simulink model "accelSim"  (R2025a)
settings: Solver=VariableStepAuto  StartTime=0.0  StopTime=5  RelTol=1e-3
InitFcn:
  | init_params();
libraries: simulink x2
settings Model: Creator=PC5  LastModifiedBy=PC5

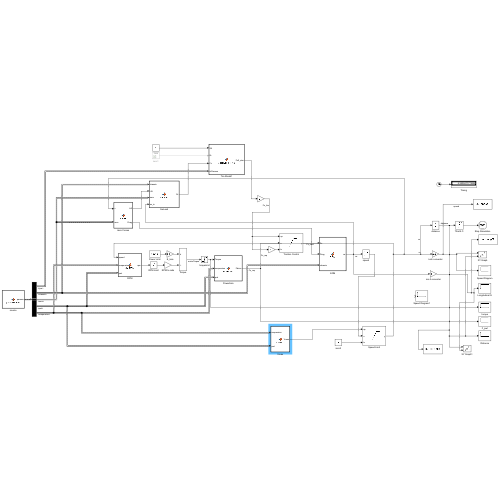
[thumbnail: Simulink's stored preview of the top-level diagram]
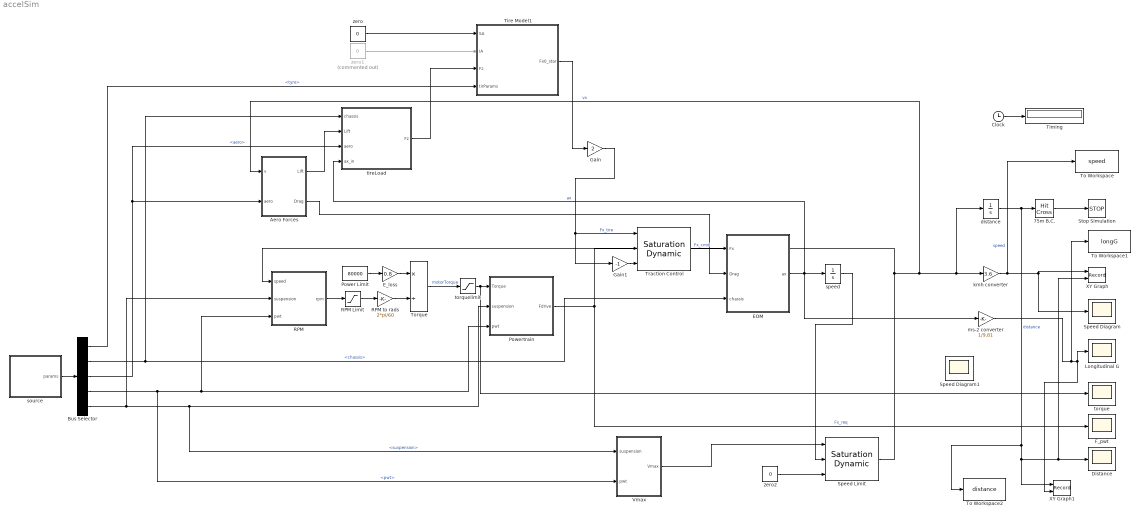
== system accelSim ==
  75m B.C. : HitCross  HitCrossingOffset=75  HitCrossingDirection=rising
  Aero Forces : MATLAB Function  TreatAsAtomicUnit=on
  Bus Selector : BusSelector  OutputSignals=tyre,chassis,aero,pwt,suspension
  Clock : Clock
  Distance : Scope
      settings: ActiveDisplayYMinimum=-1  ActiveDisplayYMaximum=1
  EOM : MATLAB Function  TreatAsAtomicUnit=on
  E_loss : Gain  Gain=0.8
  F_pwt : Scope
      settings: ActiveDisplayYMinimum=-1  ActiveDisplayYMaximum=1  DataLoggingVariableName=ScopeData4
  Gain : Gain  Gain=2
  Gain1 : Gain  Gain=-1
  Longitudinal G : Scope
      settings: Title=Longitudinal Acceleration  ActiveDisplayYMinimum=0  ActiveDisplayYMaximum=1.229  YLabel=Acceleration (G)  DataLoggingVariableName=ScopeData2
  Power Limit : Constant  Value=80000
  Powertrain : MATLAB Function  TreatAsAtomicUnit=on
  RPM : MATLAB Function  TreatAsAtomicUnit=on
  RPM Limit : Saturate  UpperLimit=10000  LowerLimit=0
  RPM to rads : Gain  Gain=2*pi/60
  Speed Diagram : Scope
      settings: ActiveDisplayYMinimum=-46.787279137521928  ActiveDisplayYMaximum=222.55498688416193
  Speed Diagram1 : Scope
      settings: ActiveDisplayYMinimum=-46.787279137521928  ActiveDisplayYMaximum=222.55498688416193  DataLoggingVariableName=ScopeData3
  Speed Limit : simulink/Discontinuities/Saturation Dynamic  OutMin=[]  OutMax=[]  OutDataTypeStr=Inherit: Same as second input  OutDataType=fixdt(1, 16)  OutScaling=2^-10  DoSatur=off
  Stop Simulation : Stop
  Timing : Display
  Tire Model1 : MATLAB Function  TreatAsAtomicUnit=on
  To Workspace : ToWorkspace  VariableName=speed  SaveFormat=Timeseries  SampleTime=-1
  To Workspace1 : ToWorkspace  VariableName=longG  SaveFormat=Timeseries  SampleTime=-1
  To Workspace2 : ToWorkspace  VariableName=distance  SaveFormat=Timeseries  SampleTime=-1
  Torque : Product  Inputs=*/  InputSameDT=on  OutMin=0  OutMax=300
  Traction Control : simulink/Discontinuities/Saturation Dynamic  OutMin=[]  OutMax=[]  OutDataTypeStr=Inherit: Same as second input  OutDataType=fixdt(1, 16)  OutScaling=2^-10  DoSatur=off
  Vmax : MATLAB Function  TreatAsAtomicUnit=on
  XY Graph : Record  NumPorts=2.0  FileSettingsInternal="{\"entries\":[{\"content\":{\"excelSettings\":{\"content\":{},\"type\":\"Streamout.ExcelSettings\"},\"parquetSettings\":{\"content\":{},\"type\":\"Streamout.ParquetSettings\"}},\"type\":\"Streamout.FileSettingStorage\",\"uuid\":\"\"}],\"packageUris\":[\"http:\\/\\/schema.mathworks.com\\/mf0\\/streamout_blocks\\/R2020a\"],\"version\":\"1.0\"}"  FrameSettings=[0, 0]  Layout=[1 1]  SignalsInternal="{\"entries\":[{\"content\":{\"signals\":[{\"content\":{\"blockPath\":[],\"dimensions\":[1],\"domain\":\"\",\"lineColor\":\"#a2142f\",\"plots\":[ 1 ],\"port\":1,\"sid\":[\"\"],\"signalID\":1,\"signalName\":\"speed\"},\"type\":\"RecordBlkView.Signal\",\"uuid\":\"\"},{\"content\":{\"blockPath\":[],\"dimensions\":[1],\"domain\":\"\",\"lineColor\":\"#139fff\",\"plots\":[ 1 ],\"port\":2,\"sid\":[\"\"],\"signalID\":2,\"signalName\":\"distance\"},\"type\":\"RecordBlkView.Signal\",\"uuid\":\"\"}]},\"type\":\"RecordBlkView.InputSignals\",\"uuid\":\"\"}],\"packageUris\":[\"http:\\/\\/schema.mathworks.com\\/mf0\\/streamout_blocks\\/R2020a\"],\"version\":\"1.0\"}"  VisualizationBindings="{\"xyplotplugin\":{\"info\":[{\"series\":[{\"bindingParametersList\":[{\"parameter\":\"X-Axis\",\"signalID\":1,\"signalName\":\"speed\"},{\"parameter\":\"Y-Axis\",\"signalID\":2,\"signalName\":\"distance\"}],\"seriesID\":0}],\"subplotID\":1}]}}"  CompatibilityTag=XY
  XY Graph1 : Record  NumPorts=2.0  FileSettingsInternal="{\"entries\":[{\"content\":{\"excelSettings\":{\"content\":{},\"type\":\"Streamout.ExcelSettings\"},\"parquetSettings\":{\"content\":{},\"type\":\"Streamout.ParquetSettings\"}},\"type\":\"Streamout.FileSettingStorage\",\"uuid\":\"\"}],\"packageUris\":[\"http:\\/\\/schema.mathworks.com\\/mf0\\/streamout_blocks\\/R2020a\"],\"version\":\"1.0\"}"  FrameSettings=[0, 0]  Layout=[1 1]  SignalsInternal="{\"entries\":[{\"content\":{\"signals\":[{\"content\":{\"blockPath\":[],\"dimensions\":[1],\"domain\":\"\",\"lineColor\":\"#a2142f\",\"plots\":[ 1 ],\"port\":1,\"sid\":[\"\"],\"signalID\":1,\"signalName\":\"distance\"},\"type\":\"RecordBlkView.Signal\",\"uuid\":\"\"},{\"content\":{\"blockPath\":[],\"dimensions\":[1],\"domain\":\"\",\"lineColor\":\"#139fff\",\"plots\":[ 1 ],\"port\":2,\"sid\":[\"\"],\"signalID\":2,\"signalName\":\"ms-2 converter\"},\"type\":\"RecordBlkView.Signal\",\"uuid\":\"\"}]},\"type\":\"RecordBlkView.InputSignals\",\"uuid\":\"\"}],\"packageUris\":[\"http:\\/\\/schema.mathworks.com\\/mf0\\/streamout_blocks\\/R2020a\"],\"version\":\"1.0\"}"  VisualizationBindings="{\"xyplotplugin\":{\"info\":[{\"series\":[{\"bindingParametersList\":[{\"parameter\":\"X-Axis\",\"signalID\":1,\"signalName\":\"distance\"},{\"parameter\":\"Y-Axis\",\"signalID\":2,\"signalName\":\"ms-2 converter\"}],\"seriesID\":0}],\"subplotID\":1}]}}"  CompatibilityTag=XY
  distance : Integrator
  kmh converter : Gain  Gain=3.6
  ms-2 converter : Gain  Gain=1/9.81
  source : MATLAB Function  TreatAsAtomicUnit=on
  speed : Integrator  LimitOutput=on  LowerSaturationLimit=0
  tireLoad : MATLAB Function  TreatAsAtomicUnit=on
  torque : Scope
      settings: ActiveDisplayYMinimum=122.82034534657527  ActiveDisplayYMaximum=241.9088505170472  DataLoggingVariableName=ScopeData5
  torquelimit : Saturate  UpperLimit=230  LowerLimit=0
  zero : Constant  Value=0
  zero1 : Constant  Commented=on  Value=0
  zero2 : Constant  Value=0
  wires:
  Aero Forces/1(Lift) -> tireLoad/2(Lift)
  Aero Forces/2(Drag) -> EOM/2(Drag)
  EOM/1(ax) -> speed/1, ms-2 converter/1, tireLoad/4(ax_in)  "ax"
  Speed Limit/1 -> distance/1, kmh converter/1, Aero Forces/1(v), RPM/1(speed)  "vx"
  Power Limit/1 -> E_loss/1
  RPM/1(rpm) -> RPM Limit/1
  distance/1 -> 75m B.C./1, To Workspace2/1, XY Graph1/1, XY Graph/2, Distance/1  "distance"
  75m B.C./1 -> Stop Simulation/1
  source/1(params) -> Bus Selector/1
  RPM Limit/1 -> RPM to rads/1
  Powertrain/1(Fdrive) -> Traction Control/2, F_pwt/1  "Fx_req"
  Gain/1 -> Gain1/1, Traction Control/1  "Fx_tire"
  Gain1/1 -> Traction Control/3
  Traction Control/1 -> EOM/1(Fx)  "Fx_cmd"
  Bus Selector/2 -> EOM/3(chassis), tireLoad/1(chassis)  "<chassis>"
  Bus Selector/3 -> Aero Forces/2(aero), tireLoad/3(aero)  "<aero>"
  Bus Selector/4 -> Vmax/2(pwt), Powertrain/3(pwt), RPM/3(pwt)  "<pwt>"
  Bus Selector/5 -> Vmax/1(suspension), Powertrain/2(suspension), RPM/2(suspension)  "<suspension>"
  kmh converter/1 -> Speed Diagram/1, XY Graph/1, To Workspace/1  "speed"
  ms-2 converter/1 -> To Workspace1/1, XY Graph1/2, Longitudinal G/1
  RPM to rads/1 -> Torque/2
  torquelimit/1 -> torque/1, Powertrain/1(Torque)
  Torque/1 -> torquelimit/1  "motorTorque"
  Clock/1 -> Timing/1
  zero/1 -> Tire Model1/1(SA)
  zero1/1 -> Tire Model1/2(IA)
  tireLoad/1(Fz) -> Tire Model1/3(Fz)
  Bus Selector/1 -> Tire Model1/4(tirParams)  "<tyre>"
  Tire Model1/1(Fx0_star) -> Gain/1
  E_loss/1 -> Torque/1
  speed/1 -> Speed Limit/2
  zero2/1 -> Speed Limit/3
  Vmax/1(Vmax) -> Speed Limit/1

== matlab function accelSim/Vmax ==
  data: Vmax output; suspension input; pwt input
% calculates aerodynamics

function Vmax  = findmaxv(suspension,pwt)

Vmax = (2*pi/60)*(pwt.max_rpm/pwt.FDR)*suspension.R;



end

== matlab function accelSim/Aero Forces ==
  data: Lift output; Drag output; v input; aero input
% calculates aerodynamics

function [Lift, Drag] = aeroF(v,aero)

Lift = 0.5*aero.farea*aero.CLs*aero.den*v^2;
Drag = 0.5*aero.farea*aero.CDs*aero.den*v^2;


end

== matlab function accelSim/tireLoad ==
  data: chassis input; Lift input; Fz output; aero input; ax_in input
function Fz = tireLoad(chassis,Lift,aero,ax_in)

mass = chassis.car+chassis.driver;
ab = aero.ab_s;
cg_h = chassis.cg_h;
wheelbase = chassis.wheelbase;

% normal load by mass
Fz = (mass*9.81)/4;
% aero downforce
AeroR = Lift*(1-ab);
% load transfer
longLT = Fz*(ax_in/9.81)*cg_h/wheelbase;
% wheel loads per wheel
Fz= Fz+AeroR/2+longLT/2;

end

== matlab function accelSim/EOM ==
  data: Fx input; ax output; Drag input; chassis input
function ax  = EOM(Fx,Drag,chassis)
ax = (Fx-Drag)/(chassis.driver+chassis.car);
end

== matlab function accelSim/RPM ==
  data: rpm output; speed input; suspension input; pwt input
function rpm = findRPM(speed,suspension,pwt)
    R = suspension.R;
    FDR = pwt.FDR;
    rpm = speed / (2*pi*R) * 60 * FDR;
end

== matlab function accelSim/Powertrain ==
  data: Torque input; Fdrive output; suspension input; pwt input
function Fdrive  = findFdrive(Torque,suspension,pwt)
R = suspension.R;
FDR = pwt.FDR;
Fdrive = FDR*Torque/R;
end

== matlab function accelSim/Tire Model1 ==
  data: SA input; IA input; Fz input; tirParams input; Fx0_star output
function Fx0_star  = accelLongForce(SA, IA, Fz, tirParams)
    % processing parameters
    Pa      = 62052.8;
    proParams = calculateParams(Fz, Pa, tirParams);

    % find peak longitudinal force
    a       = 0.05;
    d       = 0.45;
    tol     = 1e-7;
    maxIter = 5000;
    [k_star, Fx0_star, iterGold] = goldenSearchMethod(a, d, tol, maxIter, Fz, IA, tirParams, proParams);
end


function [k_star, Fx0_star, iterGold] = goldenSearchMethod(a, d, tol, maxIter, Fz, gamma, tirParams, proParams)
    % Golden ratio coefficient
    alpha = (sqrt(5) - 1) / 2;
    % Initial interior evaluation points
    b = d - alpha * (d - a);
    c = a + alpha * (d - a);
    for k = 1:maxIter
        % Evaluate magic formula longitudinal force at points b and c
        fx1 = Fx0(Fz, b, gamma, tirParams, proParams);
        fxb = fx1.Fx0;
        fx2 = Fx0(Fz, c, gamma, tirParams, proParams);
        fxc = fx2.Fx0;
        % Termination condition: search window sufficiently small
        if abs(b - a) < tol
            break
        end
        % Maximisation step (choose interval that retains the peak)
        if fxb > fxc
            % Peak lies in [a, c]
            d = c;
            c = b;
            b = d - alpha * (d - a);
        else
            % Peak lies in [b, d]
            a = b;
            b = c;
            c = a + alpha * (d - a);
        end
    end
    % Number of iterations used
    iterGold = k;
    % Select final optimum between the two interior candidates
    if fxb > fxc
        k_star   = b;
        Fx0_star = fxb;
    else
        k_star   = c;
        Fx0_star = fxc;
    end
end

function proParams = calculateParams(Fz, Pa, tirParams)
    % tirParams are fitted parameters from TIR file
    V0 = tirParams.LONGVL; %Nominal speed
    pi0	= tirParams.NOMPRES; %Nominal tyre inflation pressure
    Fz0	= tirParams.FNOMIN; %Nominal wheel load
    LFZO = tirParams.LFZO; % Scale factor of nominal (rated) load
    LMUX = tirParams.LMUX; % Scale factor of Fx peak friction coefficient
    LMUY = tirParams.LMUY; % Scale factor of Fy peak friction coefficient

    % Digressive friction factor
    % On Page 179 of the book is suggested Amu = 10, but after
    % comparing the use of the scaling factors against TNO, Amu = 1
    % was giving perfect match
    Amu = 1;
    LMUX_prime = Amu.*LMUX./(1+(Amu-1).*LMUX); % [Eqn (4.E8) Page 179 - Book]
    LMUY_prime = Amu.*LMUY./(1+(Amu-1).*LMUY); % [Eqn (4.E8) Page 179 - Book]

    % Effect of having a tire with a different nominal load
    Fz0_prime =  LFZO.*Fz0; % [Eqn (4.E1) Page 177 - Book]
    % Normalized change in vertical load
    dfz = (Fz - Fz0_prime)./Fz0_prime; % [Eqn (4.E2a) Page 177 - Book]
    % Normalized change in inflation pressure
    dpi = (Pa - pi0)./pi0; % [Eqn (4.E2b) Page 177 - Book]

    epsilon  = 1e-6;
    
    % Pack processed parameters
    proParams.LMUX_prime = LMUX_prime;
    proParams.LMUY_prime = LMUY_prime;
    proParams.Fz0_prime = Fz0_prime;
    proParams.dfz = dfz;
    proParams.dpi = dpi;
    proParams.epsilon = epsilon;
end

function fxOut = Fx0(Fz, kappa, gamma, tirParams, proParams)
    %[SCALING_COEFFICIENTS]
    LCX     = tirParams.LCX ; % Scale factor of Fx shape factor
    LEX  	= tirParams.LEX ; % Scale factor of Fx curvature factor
    LKX  	= tirParams.LKX ; % Scale factor of Fx slip stiffness
    LHX  	= tirParams.LHX ; % Scale factor of Fx horizontal shift
    LVX  	= tirParams.LVX ; % Scale factor of Fx vertical shift
    LMUX    = tirParams.LMUX ; % Scale factor of Fx peak friction coefficient
    LXAL    = tirParams.LXAL ; % Scale factor of alpha influence on Fx

    %[LONGITUDINAL_COEFFICIENTS]
    PCX1  	=  tirParams.PCX1 ; %Shape factor Cfx for longitudinal force
    PDX1  	=  tirParams.PDX1 ; %Longitudinal friction Mux at Fznom
    PDX2  	=  tirParams.PDX2 ; %Variation of friction Mux with load
    PDX3  	=  tirParams.PDX3 ; %Variation of friction Mux with camber squared
    PEX1  	=  tirParams.PEX1 ; %Longitudinal curvature Efx at Fznom
    PEX2  	=  tirParams.PEX2 ; %Variation of curvature Efx with load
    PEX3  	=  tirParams.PEX3 ; %Variation of curvature Efx with load squared
    PEX4  	=  tirParams.PEX4 ; %Factor in curvature Efx while driving
    PKX1  	=  tirParams.PKX1 ; %Longitudinal slip stiffness Kfx./Fz at Fznom
    PKX2  	=  tirParams.PKX2 ; %Variation of slip stiffness Kfx./Fz with load
    PKX3  	=  tirParams.PKX3 ; %Exponent in slip stiffness Kfx./Fz with load
    PHX1  	=  tirParams.PHX1 ; %Horizontal shift Shx at Fznom
    PHX2  	=  tirParams.PHX2 ; %Variation of shift Shx with load
    PVX1  	=  tirParams.PVX1 ; %Vertical shift Svx./Fz at Fznom
    PVX2  	=  tirParams.PVX2 ; %Variation of shift Svx./Fz with load
    PPX1  	=  tirParams.PPX1 ; %linear influence of inflation pressure on longitudinal slip stiffness
    PPX2  	=  tirParams.PPX2 ; %quadratic influence of inflation pressure on longitudinal slip stiffness
    PPX3  	=  tirParams.PPX3 ; %linear influence of inflation pressure on peak longitudinal friction
    PPX4  	=  tirParams.PPX4 ; %quadratic influence of inflation pressure on peak longitudinal friction
    
    %[PROCESSED PARAMETERS]
    dfz = proParams.dfz;
    dpi = proParams.dpi;
    LMUX_prime = proParams.LMUX_prime;
    epsilon = proParams.epsilon;

    zeta1 = 1;

    Cx = PCX1.*LCX; % (> 0) (4.E11)
    mux = (PDX1 + PDX2.*dfz).*(1 + PPX3.*dpi + PPX4.*dpi.^2).*(1 - PDX3.*gamma.^2).*LMUX; % (4.E13)
    mux(Fz==0) = 0; % Zero Fz correction
    Dx = mux.*Fz.*zeta1; % (> 0) (4.E12)
    Kxk = Fz.*(PKX1 + PKX2.*dfz).*exp(PKX3.*dfz).*(1 + PPX1.*dpi + PPX2.*dpi.^2).*LKX;  % (= BxCxDx = dFxo./dkx at kappax = 0) (= Cfk) (4.E15)
    signDx = sign(Dx);
    signDx(signDx == 0) = 1; % If [Dx = 0] then [sign(0) = 0]. This is done to avoid [Kxk / 0 = NaN] in Eqn 4.E16
    Bx = Kxk./(Cx.*Dx + epsilon.*signDx); % (4.E16) [sign(Dx) term explained on page 177]
    SHx = (PHX1 + PHX2.*dfz).*LHX; % (4.E17)
    SVx = Fz.*(PVX1 + PVX2.*dfz).*LVX.*LMUX_prime.*zeta1; % (4.E18)
    kappax = kappa + SHx; % (4.E10)
    Ex = (PEX1 + PEX2.*dfz + PEX3.*dfz.^2).*(1 - PEX4.*sign(kappax)).*LEX; % (<=1) (4.E14)
    if(any(Ex > 1))
        warning('Solver:CoeffChecks:Ex','Ex over limit (>1), Eqn(4.E14)')
        Ex(Ex > 1) = 1;
    end % if Ex > 1
    Fx0 = Dx.*sin(Cx.*atan(Bx.*kappax-Ex.*(Bx.*kappax-atan(Bx.*kappax))))+SVx; % (4.E9)
    
    % Pack pure longitudinal parameters
    fxOut.Fx0 = Fx0; % (4.E9)
    fxOut.kappax = kappax; % (4.E10)
    fxOut.Cx = Cx; % (4.E11)
    fxOut.Dx = Dx; % (4.E12)
    fxOut.mux = mux; % (4.E13)
    fxOut.Ex = Ex; % (4.E14)
    fxOut.Kxk = Kxk; % (4.E15) 
    fxOut.Bx = Bx; % (4.E16)
    fxOut.SHx = SHx; % (4.E17)
    fxOut.SVx = SVx; % (4.E18)
end

== matlab function accelSim/source ==
  data: params output Bus: ParamsBus; PARAMS parameter Bus: ParamsBus
function params = paramSource(PARAMS)
%#codegen
params = PARAMS;
end
